simulink library "determine_quadrant"  (R2022a)
settings: Solver=VariableStepAuto  StartTime=0.0  StopTime=10.0  RelTol=1e-3
settings Model: Creator=Ayaz  LastModifiedBy=lhill8
settings SolverCC: AlgebraicLoopSolver=TrustRegion
settings DebuggingCC: UnconnectedInputMsg=warning  UnconnectedOutputMsg=warning  UnconnectedLineMsg=warning  SFMachineParentedDataDiag=warning

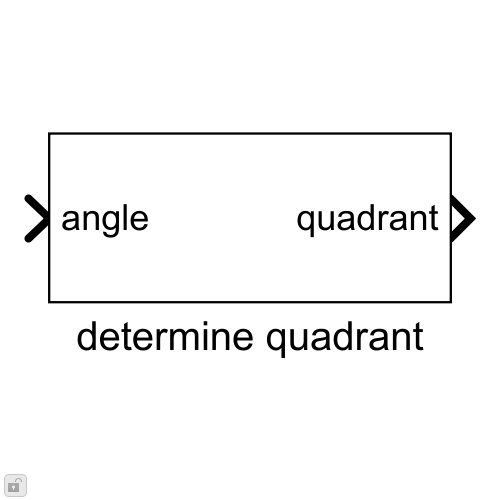
[thumbnail: Simulink's stored preview of the top-level diagram]
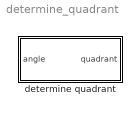
== system determine_quadrant ==
  determine quadrant : Subsystem

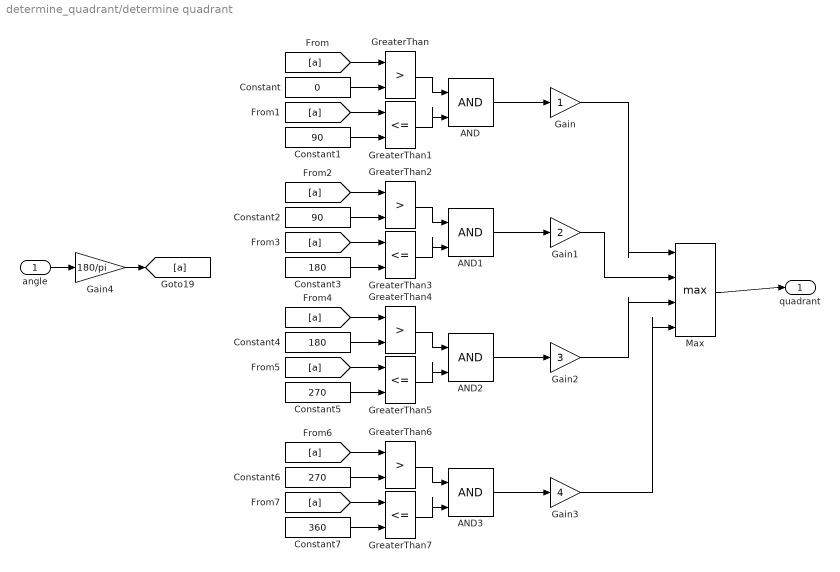
== system determine_quadrant/determine quadrant ==
  angle : Inport
  AND{,1..3} (4 alike) : Logic  IconShape=distinctive  AllPortsSameDT=off  OutDataTypeStr=boolean
  Constant : Constant  Value=0
  Constant1 : Constant  Value=90
  Constant2 : Constant  Value=90
  Constant3 : Constant  Value=180
  Constant4 : Constant  Value=180
  Constant5 : Constant  Value=270
  Constant6 : Constant  Value=270
  Constant7 : Constant  Value=360
  Gain : Gain
  Gain1 : Gain  Gain=2
  Gain2 : Gain  Gain=3
  Gain3 : Gain  Gain=4
  Gain4 : Gain  Gain=180/pi
  GreaterThan{,2,4,6} (4 alike) : RelationalOperator  Operator=>  OutDataTypeStr=boolean  RndMeth=Simplest  InputSameDT=off
  GreaterThan{1,3,5,7} (4 alike) : RelationalOperator  Operator=<=  OutDataTypeStr=boolean  RndMeth=Simplest  InputSameDT=off
  Max : MinMax  Function=max  Inputs=4
  quadrant : Outport
  wires:
  angle/1 -> Gain4/1
  [a] -> GreaterThan/1
  Constant/1 -> GreaterThan/2
  [a] -> GreaterThan1/1
  Constant1/1 -> GreaterThan1/2
  GreaterThan1/1 -> AND/2
  GreaterThan/1 -> AND/1
  GreaterThan2/1 -> AND1/1
  [a] -> GreaterThan2/1
  Constant3/1 -> GreaterThan3/2
  [a] -> GreaterThan3/1
  GreaterThan3/1 -> AND1/2
  Constant2/1 -> GreaterThan2/2
  Constant5/1 -> GreaterThan5/2
  [a] -> GreaterThan5/1
  [a] -> GreaterThan4/1
  GreaterThan5/1 -> AND2/2
  Constant4/1 -> GreaterThan4/2
  GreaterThan4/1 -> AND2/1
  GreaterThan6/1 -> AND3/1
  GreaterThan7/1 -> AND3/2
  Constant6/1 -> GreaterThan6/2
  [a] -> GreaterThan7/1
  [a] -> GreaterThan6/1
  Constant7/1 -> GreaterThan7/2
  AND/1 -> Gain/1
  AND1/1 -> Gain1/1
  AND2/1 -> Gain2/1
  AND3/1 -> Gain3/1
  Gain/1 -> Max/1
  Gain1/1 -> Max/2
  Gain2/1 -> Max/3
  Gain3/1 -> Max/4
  Max/1 -> quadrant/1
  Gain4/1 -> [a]
